simulink model "quadcopter_pd_controller"  (Simulink 8.6)
settings: Solver=VariableStepAuto  StartTime=0.0  StopTime=10  RelTol=1e-3
undefined symbols (not defined in the file or in its folder): b, g, I, k, KetaD, KetaP, KzD, KzP, l, m
settings Model: Creator=Daniel  LastModifiedBy=mgreiff
settings DataIOCC: SaveFormat=Dataset  SignalLoggingSaveFormat=Dataset
settings OptimizationCC: ExpressionDepthLimit=128
settings DebuggingCC: UnderspecifiedInitializationDetection=Simplified  MergeDetectMultiDrivingBlocksExec=error  SolverPrmCheckMsg=none  FcnCallInpInsideContextMsg=EnableAllAsError  StateNameClashWarn=none
settings HardwareCC: ProdBitPerPointer=64  ProdLargestAtomicFloat=Float  ProdIntDivRoundTo=Zero  ProdEndianess=LittleEndian  ProdWordSize=64  ProdHWDeviceType=Intel->x86-64 (Windows64)
settings GRTTargetCC: GeneratePreprocessorConditionals=Use local settings  CombineOutputUpdateFcns=on  GRTInterface=off
settings ConfigComp: CovModelRefEnable=off

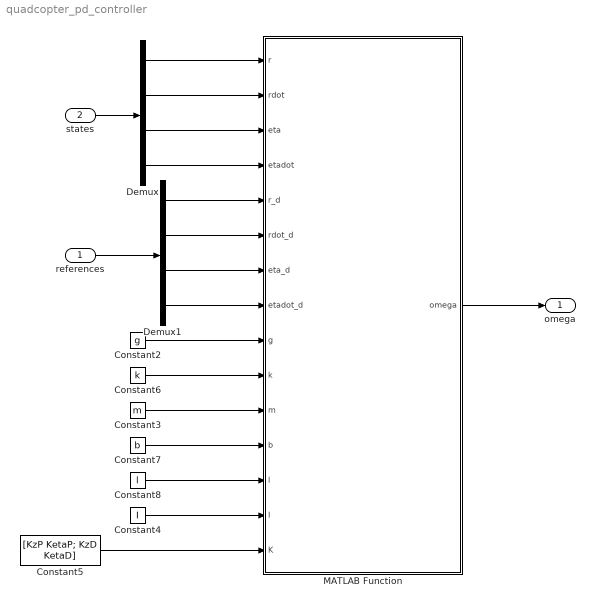
== system quadcopter_pd_controller ==
  references : Inport
  states : Inport  Port=2
  Constant2 : Constant  Value=g
  Constant3 : Constant  Value=m
  Constant4 : Constant  Value=I
  Constant5 : Constant  Value=[KzP KetaP; KzD KetaD]
  Constant6 : Constant  Value=k
  Constant7 : Constant  Value=b
  Constant8 : Constant  Value=l
  Demux : Demux  Outputs=[3,3,3,3]
  Demux1 : Demux  Outputs=[3,3,3,3]
  MATLAB Function : MATLAB Function  TreatAsAtomicUnit=on
      settings: MinAlgLoopOccurrences=on
  omega : Outport  PortDimensions=4
  wires:
  Demux/2 -> MATLAB Function/2(rdot)
  Demux/4 -> MATLAB Function/4(etadot)
  Demux1/2 -> MATLAB Function/6(rdot_d)
  Demux1/4 -> MATLAB Function/8(etadot_d)
  Constant2/1 -> MATLAB Function/9(g)
  Constant4/1 -> MATLAB Function/14(I)
  Constant3/1 -> MATLAB Function/11(m)
  Constant5/1 -> MATLAB Function/15(K)
  Constant6/1 -> MATLAB Function/10(k)
  Constant7/1 -> MATLAB Function/12(b)
  Constant8/1 -> MATLAB Function/13(l)
  MATLAB Function/1(omega) -> omega/1
  states/1 -> Demux/1
  Demux/1 -> MATLAB Function/1(r)
  Demux/3 -> MATLAB Function/3(eta)
  references/1 -> Demux1/1
  Demux1/1 -> MATLAB Function/5(r_d)
  Demux1/3 -> MATLAB Function/7(eta_d)

== matlab function MATLAB Function ==
  data: r input double; rdot input double; omega output double; eta input double; etadot input double; r_d input double; rdot_d input double; eta_d input double; etadot_d input double; g input double; k input double; m input double; b input double; l input double; I input double; K input double
function omega = copter_PD(r, rdot, eta, etadot, r_d, rdot_d, eta_d, etadot_d, g, k, m, b, l, I, K)
    KzP = K(1,1); KetaP = K(1,2:4)';
    KzD = K(2,1); KetaD = K(2,2:4)';
    
    phi = eta(1); theta = eta(2); psi = eta(3);
    
    T = m/(cos(phi)*cos(theta)) * (g + KzD * (rdot_d(3) - rdot(3)) + KzP * (r_d(3) - r(3)));
    tau = diag(I) * (KetaD .* (etadot_d - etadot) + KetaP .* (eta_d - eta));
    tau_phi = tau(1); tau_theta = tau(2); tau_psi = tau(3);
    
    
    w1sq = T/(4*k) - tau_theta/(2*k*l) - tau_psi / (4*b);
    w2sq = T/(4*k) - tau_phi/(2*k*l) + tau_psi / (4*b);
    w3sq = T/(4*k) + tau_theta/(2*k*l) - tau_psi / (4*b);
    w4sq = T/(4*k) + tau_phi/(2*k*l) + tau_psi / (4*b);
    
    omega = sqrt(max([w1sq w2sq w3sq w4sq]', 0));
end
